simulink model "Control_try"  (R2021b)
settings: Solver=VariableStepAuto  StartTime=0.0  StopTime=inf  RelTol=1e-3
undefined symbols (not defined in the file or in its folder): DiscIntNeverNeededParam
libraries: mobileRoboticsLib x25, simulink_extras x1
(part 1 of 2)
settings Model: Creator=its_ghani  LastModifiedBy=nitis

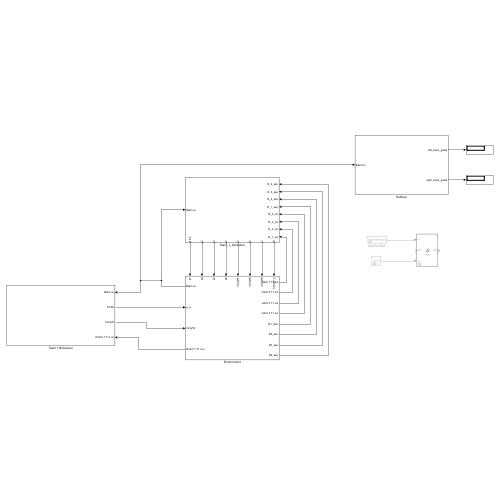
[thumbnail: Simulink's stored preview of the top-level diagram]
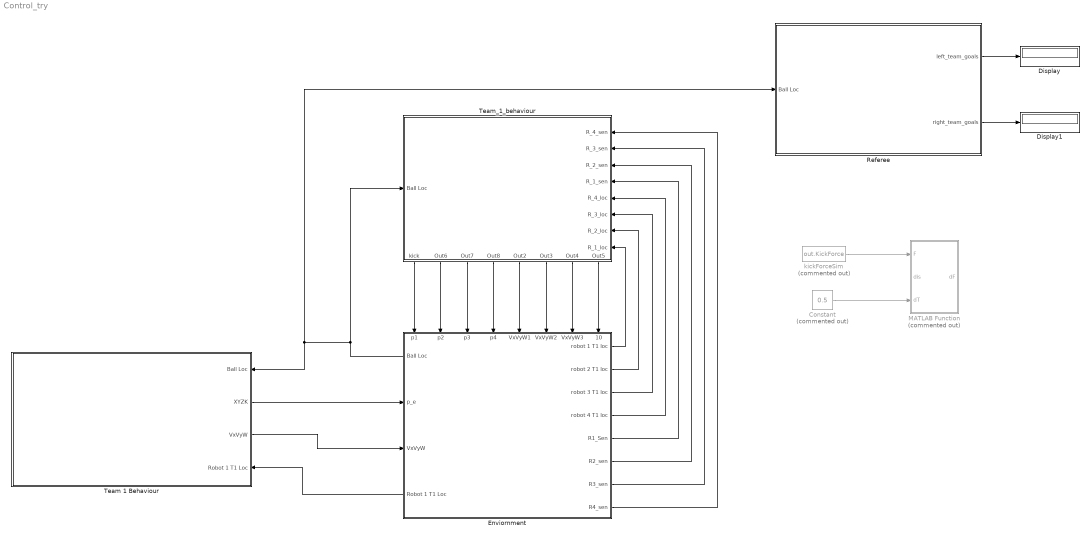
== system Control_try ==
  Constant : Constant  Commented=on  Value=0.5
  Display : Display
  Display1 : Display
  Enviornment : Subsystem
      settings: PortSchema="{\"entries\":[{\"content\":{\"sides\":[{\"content\":{\"connectorIds\":[\"Out9\",\"In1\",\"In2\",\"Out10\"]},\"type\":\"ConnectorPlacement.EquallySpacedRectSide\",\"uuid\":\"bfc4f995-18bb-40a5-813e-439d500b4bf9\"},{\"content\":{\"connectorIds\":[\"Out1\",\"Out2\",\"Out3\",\"Out4\",\"Out5\",\"Out6\",\"Out7\",\"Out8\"],\"side\":\"RIGHT\"},\"type\":\"ConnectorPlacement.EquallySpacedRectSide\",\"uuid\":\"3fb6b8a6-16df-4a59-8ba5-6321e26d1fdd\"},{\"content\":{\"connectorIds\":[\"In3\",\"In4\",\"In5\",\"In6\",\"In7\",\"In8\",\"In9\",\"In10\"],\"side\":\"TOP\"},\"type\":\"ConnectorPlacement.EquallySpacedRectSide\",\"uuid\":\"a9e4cd1b-3afe-4395-99fa-15aef12a4070\"}]},\"type\":\"ConnectorPlacement.EquallySpacedConnector\",\"uuid\":\"a6ca697e-fe67-43ac-b669-91f3e6c836c9\"}],\"packageUris\":[\"http://schema.mathworks.com/mf0/Connector/R2020b\"],\"version\":\"1.0\"}"
  MATLAB Function : MATLAB Function  Commented=on  TreatAsAtomicUnit=on
  Referee : Subsystem
  Team 1 Behaviour : Subsystem
      settings: PortSchema="{\"entries\":[{\"content\":{\"sides\":[{\"content\":{\"connectorIds\":[]},\"type\":\"ConnectorPlacement.EquallySpacedRectSide\",\"uuid\":\"be901545-21b9-45e5-bac5-a8cb9027aef5\"},{\"content\":{\"connectorIds\":[\"In1\",\"Out1\",\"Out2\",\"In2\"],\"side\":\"RIGHT\"},\"type\":\"ConnectorPlacement.EquallySpacedRectSide\",\"uuid\":\"b7c1eb84-2f14-4c7f-a74c-d56efbe0743e\"},{\"content\":{\"connectorIds\":[],\"side\":\"TOP\"},\"type\":\"ConnectorPlacement.EquallySpacedRectSide\",\"uuid\":\"aca41723-ed3f-4bd2-8fc1-457d075e3460\"}]},\"type\":\"ConnectorPlacement.EquallySpacedConnector\",\"uuid\":\"e10e22f1-c8f0-4dfc-85d2-4ba01528372d\"}],\"packageUris\":[\"http://schema.mathworks.com/mf0/Connector/R2020b\"],\"version\":\"1.0\"}"
  Team_1_behaviour : Subsystem
      settings: PortSchema="{\"entries\":[{\"content\":{\"sides\":[{\"content\":{\"connectorIds\":[\"In1\"]},\"type\":\"ConnectorPlacement.EquallySpacedRectSide\",\"uuid\":\"3d238569-03e8-47ba-93af-d09e13fdb2d4\"},{\"content\":{\"connectorIds\":[\"In2\",\"In3\",\"In4\",\"In5\",\"In6\",\"In7\",\"In8\",\"In9\"],\"side\":\"RIGHT\"},\"type\":\"ConnectorPlacement.EquallySpacedRectSide\",\"uuid\":\"12d8afb4-4727-4f82-8566-507ab080c6de\"},{\"content\":{\"connectorIds\":[],\"side\":\"TOP\"},\"type\":\"ConnectorPlacement.EquallySpacedRectSide\",\"uuid\":\"c52fa7ec-51b7-43be-84ca-6ce417c012c7\"},{\"content\":{\"connectorIds\":[\"Out1\",\"Out2\",\"Out3\",\"Out4\",\"Out5\",\"Out6\",\"Out7\",\"Out8\"],\"side\":\"BOTTOM\"},\"type\":\"ConnectorPlacement.EquallySpacedRectSide\",\"uuid\":\"1ba4ac49-8e90-4b3f-8374-c14756940453\"}]},\"type\":\"ConnectorPlacement.EquallySpacedConnector\",\"uuid\":\"883bb5df-d6b2-498f-94a4-3b94e28c6a8f\"}],\"packageUris\":[\"http://schema.mathworks.com/mf0/Connector/R2020b\"],\"version\":\"1.0\"}"
  kickForceSim : FromWorkspace  Commented=on  VariableName=out.KickForce
  wires:
  Enviornment/9(Ball Loc) -> Team_1_behaviour/1(Ball Loc), Referee/1(Ball Loc), Team 1 Behaviour/1(Ball Loc)
  Team 1 Behaviour/1(XYZK) -> Enviornment/1(p_e)
  Referee/2(right_team_goals) -> Display1/1
  Referee/1(left_team_goals) -> Display/1
  Team 1 Behaviour/2(VxVyW) -> Enviornment/2(VxVyW)
  Enviornment/10(Robot 1 T1 Loc) -> Team 1 Behaviour/2(Robot 1 T1 Loc)
  Team_1_behaviour/5(Out2) -> Enviornment/7(VxVyW1)
  Team_1_behaviour/6(Out3) -> Enviornment/8(VxVyW2)
  Team_1_behaviour/7(Out4) -> Enviornment/9(VxVyW3)
  Team_1_behaviour/8(Out5) -> Enviornment/10(VxVyW_4)
  Enviornment/1(robot 1 T1 loc) -> Team_1_behaviour/9(R_1_loc)
  Enviornment/2(robot 2 T1 loc) -> Team_1_behaviour/8(R_2_loc)
  Enviornment/3(robot 3 T1 loc) -> Team_1_behaviour/7(R_3_loc)
  Enviornment/4(robot 4 T1 loc) -> Team_1_behaviour/6(R_4_loc)
  Enviornment/5(R1_Sen) -> Team_1_behaviour/5(R_1_sen)
  Enviornment/6(R2_sen) -> Team_1_behaviour/4(R_2_sen)
  Enviornment/7(R3_sen) -> Team_1_behaviour/3(R_3_sen)
  Enviornment/8(R4_sen) -> Team_1_behaviour/2(R_4_sen)
  Team_1_behaviour/1(kick) -> Enviornment/3(p1)
  Team_1_behaviour/2(Out6) -> Enviornment/4(p2)
  Team_1_behaviour/3(Out7) -> Enviornment/5(p3)
  Team_1_behaviour/4(Out8) -> Enviornment/6(p4)
  kickForceSim/1 -> MATLAB Function/1(F)
  Constant/1 -> MATLAB Function/3(dT)

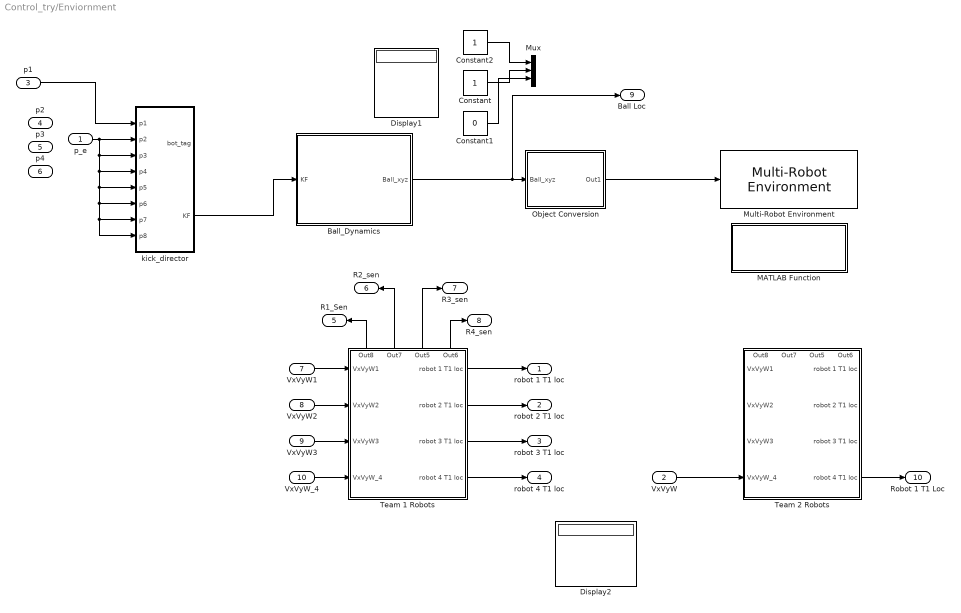
== system Control_try/Enviornment ==
  p_e : Inport
  VxVyW : Inport  Port=2
  p1 : Inport  Port=3
  p2 : Inport  Port=4
  p3 : Inport  Port=5
  p4 : Inport  Port=6
  VxVyW1 : Inport  Port=7
  VxVyW2 : Inport  Port=8
  VxVyW3 : Inport  Port=9
  VxVyW_4 : Inport  Port=10
  "\tTeam 1 Robots" : Subsystem
      settings: PortSchema="{\"entries\":[{\"content\":{\"sides\":[{\"content\":{\"connectorIds\":[\"In1\",\"In2\",\"In3\",\"In4\"]},\"type\":\"ConnectorPlacement.EquallySpacedRectSide\",\"uuid\":\"e759642f-fbca-4f1e-b212-daca2c4962f8\"},{\"content\":{\"connectorIds\":[\"Out1\",\"Out2\",\"Out3\",\"Out4\"],\"side\":\"RIGHT\"},\"type\":\"ConnectorPlacement.EquallySpacedRectSide\",\"uuid\":\"6e1699fa-b246-4758-836f-1d4c98857b70\"},{\"content\":{\"connectorIds\":[\"Out5\",\"Out6\",\"Out7\",\"Out8\"],\"side\":\"TOP\"},\"type\":\"ConnectorPlacement.EquallySpacedRectSide\",\"uuid\":\"c1cf0a96-808a-4241-9d01-181cc4ce2a4d\"},{\"content\":{\"connectorIds\":[],\"side\":\"BOTTOM\"},\"type\":\"ConnectorPlacement.EquallySpacedRectSide\",\"uuid\":\"1a7f648f-16d5-4a09-b479-d6590fa53252\"}]},\"type\":\"ConnectorPlacement.EquallySpacedConnector\",\"uuid\":\"5972ed04-ecdd-4117-bf5d-456318b5c4b8\"}],\"packageUris\":[\"http://schema.mathworks.com/mf0/Connector/R2020b\"],\"version\":\"1.0\"}"
  "\tTeam 2 Robots" : Subsystem
      settings: PortSchema="{\"entries\":[{\"content\":{\"sides\":[{\"content\":{\"connectorIds\":[\"In1\",\"In2\",\"In3\",\"In4\"]},\"type\":\"ConnectorPlacement.EquallySpacedRectSide\",\"uuid\":\"e759642f-fbca-4f1e-b212-daca2c4962f8\"},{\"content\":{\"connectorIds\":[\"Out1\",\"Out2\",\"Out3\",\"Out4\"],\"side\":\"RIGHT\"},\"type\":\"ConnectorPlacement.EquallySpacedRectSide\",\"uuid\":\"6e1699fa-b246-4758-836f-1d4c98857b70\"},{\"content\":{\"connectorIds\":[\"Out5\",\"Out6\",\"Out7\",\"Out8\"],\"side\":\"TOP\"},\"type\":\"ConnectorPlacement.EquallySpacedRectSide\",\"uuid\":\"c1cf0a96-808a-4241-9d01-181cc4ce2a4d\"},{\"content\":{\"connectorIds\":[],\"side\":\"BOTTOM\"},\"type\":\"ConnectorPlacement.EquallySpacedRectSide\",\"uuid\":\"1a7f648f-16d5-4a09-b479-d6590fa53252\"}]},\"type\":\"ConnectorPlacement.EquallySpacedConnector\",\"uuid\":\"5972ed04-ecdd-4117-bf5d-456318b5c4b8\"}],\"packageUris\":[\"http://schema.mathworks.com/mf0/Connector/R2020b\"],\"version\":\"1.0\"}"
  Ball_Dynamics : Subsystem
  Constant : Constant
  Constant1 : Constant  Value=0
  Constant2 : Constant
  Display1 : Display
  Display2 : Display
  MATLAB Function : MATLAB Function  TreatAsAtomicUnit=on
  Multi-Robot Environment : mobileRoboticsLib/Environments/Multi-Robot Environment  numRobots=8  showWaypoints=off  showObjects=on  objectColors=[1 0 0;0 1 0;0 0 1]  objectMarkers='c'  showRobotIds=on  plotSensorLines=on
      settings: SourceProductName=Mobile Robotics Simulation Toolbox
  Mux : Mux  Inputs=3
  Object Conversion : Subsystem
  kick_director : Subsystem
  robot 1 T1 loc : Outport
  robot 2 T1 loc : Outport  Port=2
  robot 3 T1 loc : Outport  Port=3
  robot 4 T1 loc : Outport  Port=4
  R1_Sen : Outport  Port=5
  R2_sen : Outport  Port=6
  R3_sen : Outport  Port=7
  R4_sen : Outport  Port=8
  Ball Loc : Outport  Port=9
  Robot 1 T1 Loc : Outport  Port=10
  wires:
  "\tTeam 1 Robots"/1(robot 1 T1 loc) -> robot 1 T1 loc/1
  Object Conversion/1(Out1) -> Multi-Robot Environment/1
  "\tTeam 1 Robots"/2(robot 2 T1 loc) -> robot 2 T1 loc/1
  "\tTeam 1 Robots"/3(robot 3 T1 loc) -> robot 3 T1 loc/1
  "\tTeam 1 Robots"/4(robot 4 T1 loc) -> robot 4 T1 loc/1
  VxVyW1/1 -> "\tTeam 1 Robots"/1(VxVyW1)
  VxVyW3/1 -> "\tTeam 1 Robots"/3(VxVyW3)
  VxVyW_4/1 -> "\tTeam 1 Robots"/4(VxVyW_4)
  "\tTeam 1 Robots"/5(Out8) -> R1_Sen/1
  "\tTeam 1 Robots"/6(Out7) -> R2_sen/1
  "\tTeam 1 Robots"/7(Out5) -> R3_sen/1
  "\tTeam 1 Robots"/8(Out6) -> R4_sen/1
  p_e/1 -> kick_director/4(p4), kick_director/5(p5), kick_director/6(p6), kick_director/7(p7), kick_director/8(p8), kick_director/3(p3), kick_director/2(p2)
  p1/1 -> kick_director/1(p1)
  VxVyW2/1 -> "\tTeam 1 Robots"/2(VxVyW2)
  "\tTeam 2 Robots"/4(robot 4 T1 loc) -> Robot 1 T1 Loc/1
  VxVyW/1 -> "\tTeam 2 Robots"/4(VxVyW_4)
  kick_director/2(KF) -> Ball_Dynamics/1(KF)
  Constant2/1 -> Mux/1
  Constant/1 -> Mux/2
  Constant1/1 -> Mux/3
  Ball_Dynamics/1(Ball_xyz) -> Ball Loc/1, Object Conversion/1(Ball_xyz)

== system Control_try/Referee ==
  Ball Loc : Inport
  Corner : Stateflow chart  TreatAsAtomicUnit=on
  Demux : Demux  Outputs=3
  Display2 : Display
  GOAL : Stateflow chart  TreatAsAtomicUnit=on
  Penelty : Stateflow chart  TreatAsAtomicUnit=on
  Throwin : Stateflow chart  TreatAsAtomicUnit=on
  left_team_goals : Outport
  right_team_goals : Outport  Port=2
  wires:
  Ball Loc/1 -> Display2/1, Demux/1
  Demux/1 -> Throwin/1(X), GOAL/1(X)
  Demux/2 -> Throwin/2(Y), GOAL/2(Y)
  Demux/3 -> GOAL/3(Z)
  GOAL/1(left_team_goal) -> left_team_goals/1
  GOAL/2(right_team_goal) -> right_team_goals/1

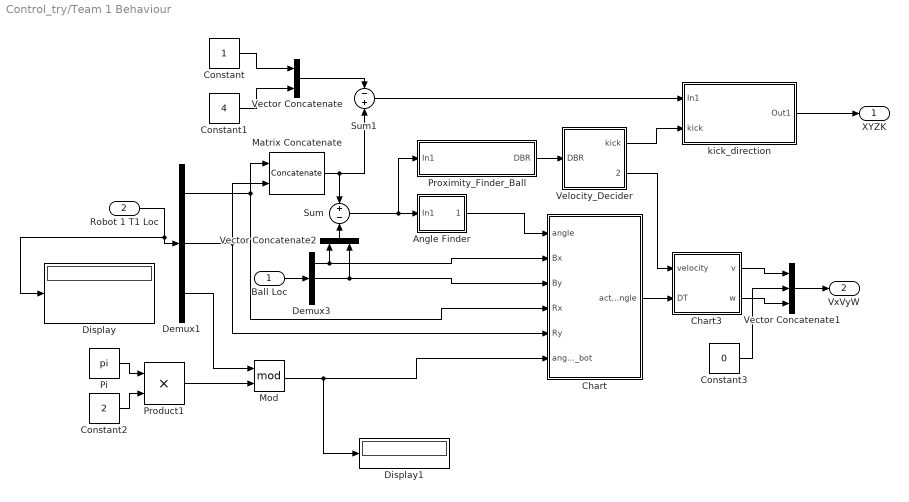
== system Control_try/Team 1 Behaviour ==
  Ball Loc : Inport
  Robot 1 T1 Loc : Inport  Port=2
  Angle Finder : Subsystem
  Chart : Stateflow chart  TreatAsAtomicUnit=on
      settings: PortSchema="{\"entries\":[{\"content\":{\"sides\":[{\"content\":{\"connectorIds\":[\"In5\",\"In1\",\"In2\",\"In3\",\"In4\",\"In6\"]},\"type\":\"ConnectorPlacement.EquallySpacedRectSide\",\"uuid\":\"cd25ea97-6441-4246-83f2-eec847899c89\"},{\"content\":{\"connectorIds\":[\"Out1\"],\"side\":\"RIGHT\"},\"type\":\"ConnectorPlacement.EquallySpacedRectSide\",\"uuid\":\"ef7d77a7-1549-4474-8b84-35bb8af5d0e7\"},{\"content\":{\"connectorIds\":[],\"side\":\"TOP\"},\"type\":\"ConnectorPlacement.EquallySpacedRectSide\",\"uuid\":\"0f0ce596-3061-42ac-890a-62bc4f21ac3e\"},{\"content\":{\"connectorIds\":[],\"side\":\"BOTTOM\"},\"type\":\"ConnectorPlacement.EquallySpacedRectSide\",\"uuid\":\"682b3de5-e999-4954-b7ff-f16ecbf9ea8f\"}]},\"type\":\"ConnectorPlacement.EquallySpacedConnector\",\"uuid\":\"15dca8e2-6a60-4a0d-80a5-3c295a61c828\"}],\"packageUris\":[\"http://schema.mathworks.com/mf0/Connector/R2020b\"],\"version\":\"1.0\"}"
  Chart3 : Stateflow chart  TreatAsAtomicUnit=on
  Constant : Constant
  Constant1 : Constant  Value=4
  Constant2 : Constant  Value=2
  Constant3 : Constant  Value=0
  Demux1 : Demux  Outputs=3
  Demux3 : Demux  Outputs=3
  Display : Display
  Display1 : Display
  Matrix Concatenate : Concatenate  Mode=Multidimensional array  ConcatenateDimension=2
  Mod : Math  Operator=mod  SaturateOnIntegerOverflow=on
  Pi : Constant  Value=pi  OutDataTypeStr=Inherit: Inherit via back propagation
  Product1 : Product
  Proximity_Finder_Ball : Subsystem
  Sum : Sum  Inputs=+-
  Sum1 : Sum  Inputs=-+
  Vector Concatenate : Concatenate
  Vector Concatenate1 : Concatenate  NumInputs=3
  Vector Concatenate2 : Concatenate
  Velocity_Decider : Stateflow chart  TreatAsAtomicUnit=on
  kick_direction : Subsystem
  XYZK : Outport
  VxVyW : Outport  Port=2
  wires:
  Ball Loc/1 -> Demux3/1
  Sum/1 -> Proximity_Finder_Ball/1(In1), Angle Finder/1(In1)
  Robot 1 T1 Loc/1 -> Display/1, Demux1/1
  Demux1/1 -> Matrix Concatenate/1, Chart/3(Rx)
  Demux1/2 -> Matrix Concatenate/2, Chart/4(Ry)
  Matrix Concatenate/1 -> Sum1/2, Sum/1
  Demux3/2 -> Vector Concatenate2/2, Chart/2(By)
  Demux3/1 -> Vector Concatenate2/1, Chart/1(Bx)
  Demux1/3 -> Mod/1
  Pi/1 -> Product1/1
  Constant2/1 -> Product1/2
  Product1/1 -> Mod/2
  Chart/1(actual_angle) -> Chart3/2(DT)
  Mod/1 -> Display1/1, Chart/6(angle_bot)
  Angle Finder/1(angle) -> Chart/5(angle)
  Proximity_Finder_Ball/1(DBR) -> Velocity_Decider/1(DBR)
  Velocity_Decider/2(velocity) -> Chart3/1(velocity)
  Constant/1 -> Vector Concatenate/1
  Constant1/1 -> Vector Concatenate/2
  Vector Concatenate/1 -> Sum1/1
  Sum1/1 -> kick_direction/1(In1)
  Velocity_Decider/1(kick) -> kick_direction/2(kick)
  kick_direction/1(Out1) -> XYZK/1
  Chart3/1(v) -> Vector Concatenate1/1
  Chart3/2(w) -> Vector Concatenate1/3
  Constant3/1 -> Vector Concatenate1/2
  Vector Concatenate1/1 -> VxVyW/1
  Vector Concatenate2/1 -> Sum/2

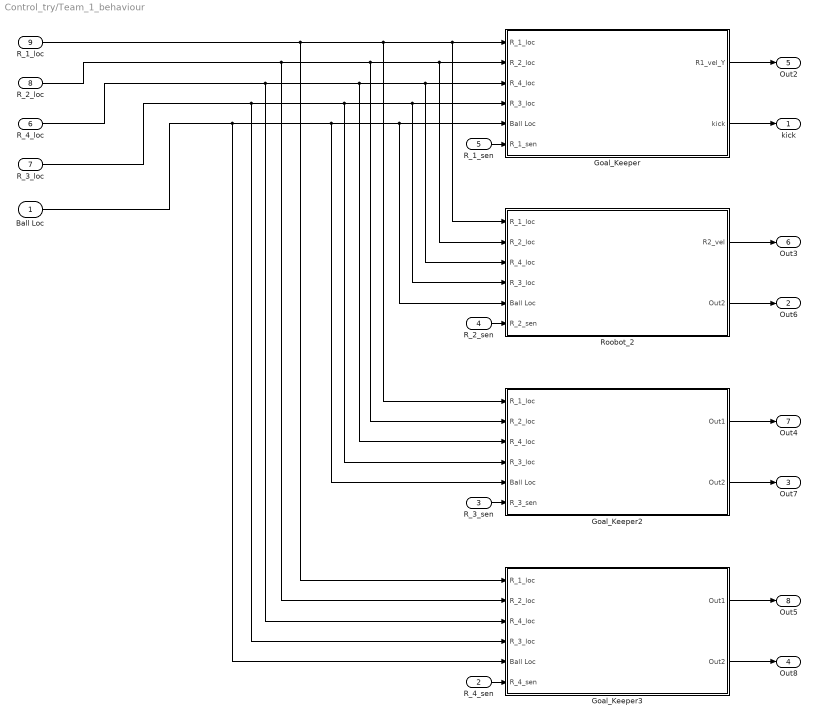
== system Control_try/Team_1_behaviour ==
  Ball Loc : Inport
  R_4_sen : Inport  Port=2
  R_3_sen : Inport  Port=3
  R_2_sen : Inport  Port=4
  R_1_sen : Inport  Port=5
  R_4_loc : Inport  Port=6
  R_3_loc : Inport  Port=7
  R_2_loc : Inport  Port=8
  R_1_loc : Inport  Port=9
  Goal_Keeper : Subsystem
  Goal_Keeper2 : Subsystem
  Goal_Keeper3 : Subsystem
  Roobot_2 : Subsystem
  kick : Outport
  Out6 : Outport  Port=2
  Out7 : Outport  Port=3
  Out8 : Outport  Port=4
  Out2 : Outport  Port=5
  Out3 : Outport  Port=6
  Out4 : Outport  Port=7
  Out5 : Outport  Port=8
  wires:
  Goal_Keeper/1(R1_vel_Y) -> Out2/1
  R_1_sen/1 -> Goal_Keeper/6(R_1_sen)
  R_1_loc/1 -> Goal_Keeper3/1(R_1_loc), Goal_Keeper2/1(R_1_loc), Roobot_2/1(R_1_loc), Goal_Keeper/1(R_1_loc)
  R_2_loc/1 -> Goal_Keeper3/2(R_2_loc), Goal_Keeper2/2(R_2_loc), Roobot_2/2(R_2_loc), Goal_Keeper/2(R_2_loc)
  R_4_loc/1 -> Goal_Keeper3/3(R_4_loc), Goal_Keeper2/3(R_4_loc), Roobot_2/3(R_4_loc), Goal_Keeper/3(R_4_loc)
  R_3_loc/1 -> Goal_Keeper3/4(R_3_loc), Goal_Keeper2/4(R_3_loc), Roobot_2/4(R_3_loc), Goal_Keeper/4(R_3_loc)
  Ball Loc/1 -> Goal_Keeper3/5(Ball Loc), Goal_Keeper2/5(Ball Loc), Roobot_2/5(Ball Loc), Goal_Keeper/5(Ball Loc)
  R_2_sen/1 -> Roobot_2/6(R_2_sen)
  R_3_sen/1 -> Goal_Keeper2/6(R_3_sen)
  R_4_sen/1 -> Goal_Keeper3/6(R_4_sen)
  Roobot_2/1(R2_vel) -> Out3/1
  Goal_Keeper2/1(Out1) -> Out4/1
  Goal_Keeper3/1(Out1) -> Out5/1
  Goal_Keeper/2(kick) -> kick/1
  Roobot_2/2(Out2) -> Out6/1
  Goal_Keeper2/2(Out2) -> Out7/1
  Goal_Keeper3/2(Out2) -> Out8/1

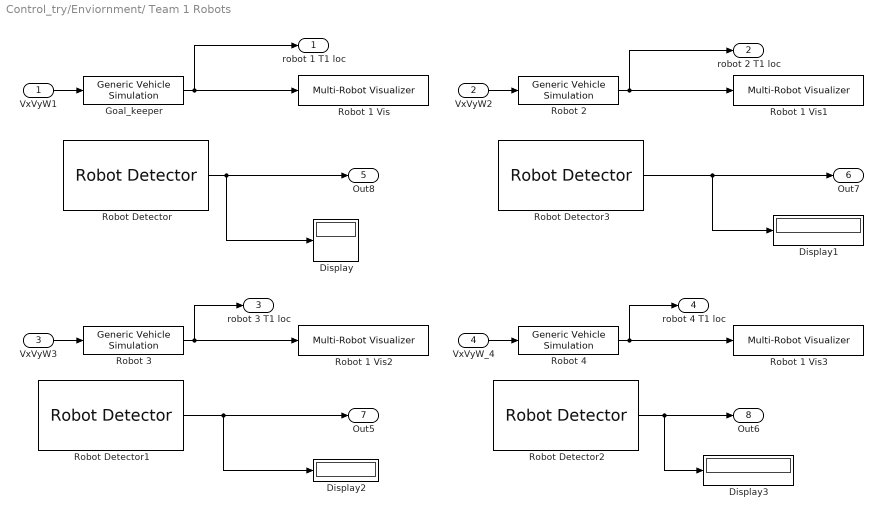
== system Control_try/Enviornment/	Team 1 Robots ==
  VxVyW1 : Inport
  VxVyW2 : Inport  Port=2
  VxVyW3 : Inport  Port=3
  VxVyW_4 : Inport  Port=4
  Display{,1..3} (4 alike) : Display
  Goal_keeper : mobileRoboticsLib/Utilities/Generic Vehicle Simulation  initX=1.5  initY=4  initAngle=0  Ts=0.05
      settings: SourceProductName=Mobile Robotics Simulation Toolbox
  Robot 1 Vis : mobileRoboticsLib/Environments/Multi-Robot Visualizer  idx=1  radius=0.5  robotColor=[0 0 1]  showTraj=on  hasLidar=off  sensorOffset=[0,0]  scanAngles=[-pi/4, 0, pi/4]  hasObjDetector=off  objDetectorOffset=[0,0]  objDetectorAngle=0  objDetectorFOV=pi/3  objDetectorMaxRange=5
      settings: SourceProductName=Mobile Robotics Simulation Toolbox
  Robot 1 Vis1 : mobileRoboticsLib/Environments/Multi-Robot Visualizer  idx=2  radius=0.5  robotColor=[0 0 1]  showTraj=on  hasLidar=off  sensorOffset=[0,0]  scanAngles=[-pi/4, 0, pi/4]  hasObjDetector=off  objDetectorOffset=[0,0]  objDetectorAngle=0  objDetectorFOV=pi/3  objDetectorMaxRange=5
      settings: SourceProductName=Mobile Robotics Simulation Toolbox
  Robot 1 Vis2 : mobileRoboticsLib/Environments/Multi-Robot Visualizer  idx=3  radius=0.5  robotColor=[0 0 1]  showTraj=on  hasLidar=off  sensorOffset=[0,0]  scanAngles=[-pi/4, 0, pi/4]  hasObjDetector=off  objDetectorOffset=[0,0]  objDetectorAngle=0  objDetectorFOV=pi/3  objDetectorMaxRange=5
      settings: SourceProductName=Mobile Robotics Simulation Toolbox
  Robot 1 Vis3 : mobileRoboticsLib/Environments/Multi-Robot Visualizer  idx=4  radius=0.5  robotColor=[0 0 1]  showTraj=on  hasLidar=off  sensorOffset=[0,0]  scanAngles=[-pi/4, 0, pi/4]  hasObjDetector=off  objDetectorOffset=[0,0]  objDetectorAngle=0  objDetectorFOV=pi/3  objDetectorMaxRange=5
      settings: SourceProductName=Mobile Robotics Simulation Toolbox
  Robot 2 : mobileRoboticsLib/Utilities/Generic Vehicle Simulation  initX=3.25  initY=2.5  initAngle=0  Ts=0.05
      settings: SourceProductName=Mobile Robotics Simulation Toolbox
  Robot 3 : mobileRoboticsLib/Utilities/Generic Vehicle Simulation  initX=3.25  initY=5.5  initAngle=0  Ts=0.05
      settings: SourceProductName=Mobile Robotics Simulation Toolbox
  Robot 4 : mobileRoboticsLib/Utilities/Generic Vehicle Simulation  initX=5.25  initY=4.25  initAngle=0  Ts=0.05
      settings: SourceProductName=Mobile Robotics Simulation Toolbox
  Robot Detector : mobileRoboticsLib/Environments/Robot Detector  robotIdx=1  sensorOffset=[ 0, 0 ]  sensorAngle=0  fieldOfView=pi/3  maxRange=3  maxDetections=7  sampleTime=0.1
      settings: SourceProductName=Mobile Robotics Simulation Toolbox
  Robot Detector1 : mobileRoboticsLib/Environments/Robot Detector  robotIdx=3  sensorOffset=[ 0, 0 ]  sensorAngle=0  fieldOfView=pi/3  maxRange=1.5  maxDetections=7  sampleTime=0.1
      settings: SourceProductName=Mobile Robotics Simulation Toolbox
  Robot Detector2 : mobileRoboticsLib/Environments/Robot Detector  robotIdx=4  sensorOffset=[ 0, 0 ]  sensorAngle=0  fieldOfView=pi/3  maxRange=1.5  maxDetections=7  sampleTime=0.1
      settings: SourceProductName=Mobile Robotics Simulation Toolbox
  Robot Detector3 : mobileRoboticsLib/Environments/Robot Detector  robotIdx=2  sensorOffset=[ 0, 0 ]  sensorAngle=0  fieldOfView=pi/3  maxRange=1.5  maxDetections=7  sampleTime=0.1
      settings: SourceProductName=Mobile Robotics Simulation Toolbox
  robot 1 T1 loc : Outport
  robot 2 T1 loc : Outport  Port=2
  robot 3 T1 loc : Outport  Port=3
  robot 4 T1 loc : Outport  Port=4
  Out8 : Outport  Port=5
  Out7 : Outport  Port=6
  Out5 : Outport  Port=7
  Out6 : Outport  Port=8
  wires:
  Goal_keeper/1 -> robot 1 T1 loc/1, Robot 1 Vis/1
  VxVyW1/1 -> Goal_keeper/1
  VxVyW2/1 -> Robot 2/1
  Robot 2/1 -> robot 2 T1 loc/1, Robot 1 Vis1/1
  Robot 3/1 -> Robot 1 Vis2/1, robot 3 T1 loc/1
  VxVyW3/1 -> Robot 3/1
  VxVyW_4/1 -> Robot 4/1
  Robot 4/1 -> robot 4 T1 loc/1, Robot 1 Vis3/1
  Robot Detector3/1 -> Out7/1, Display1/1
  Robot Detector1/1 -> Out5/1, Display2/1
  Robot Detector2/1 -> Out6/1, Display3/1
  Robot Detector/1 -> Display/1, Out8/1

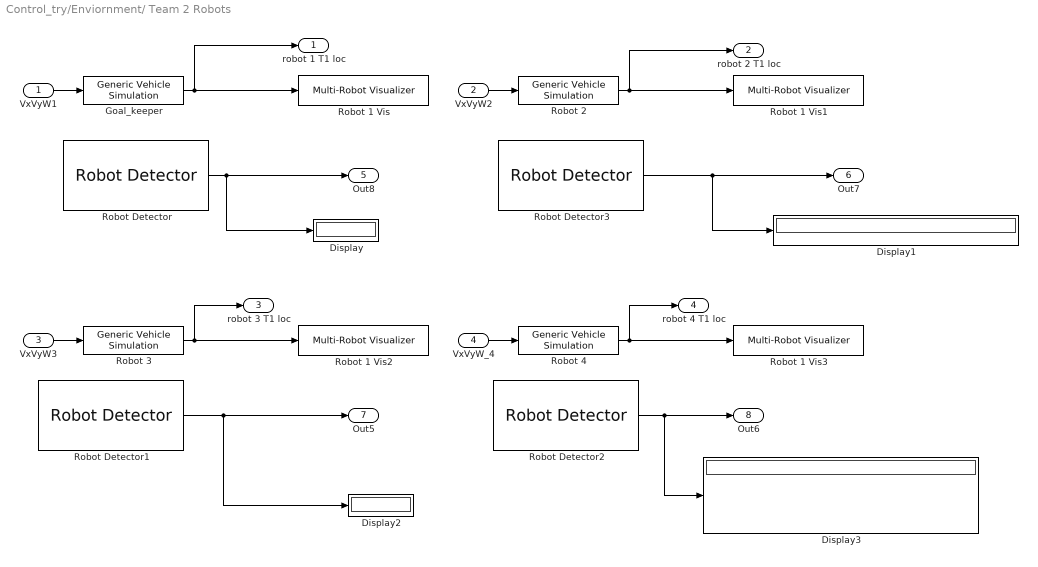
== system Control_try/Enviornment/	Team 2 Robots ==
  VxVyW1 : Inport
  VxVyW2 : Inport  Port=2
  VxVyW3 : Inport  Port=3
  VxVyW_4 : Inport  Port=4
  Display{,1..3} (4 alike) : Display
  Goal_keeper : mobileRoboticsLib/Utilities/Generic Vehicle Simulation  initX=9.5  initY=4  initAngle=pi  Ts=0.05
      settings: SourceProductName=Mobile Robotics Simulation Toolbox
  Robot 1 Vis : mobileRoboticsLib/Environments/Multi-Robot Visualizer  idx=5  radius=0.5  robotColor=[1 0 0]  showTraj=on  hasLidar=off  sensorOffset=[0,0]  scanAngles=[-pi/4, 0, pi/4]  hasObjDetector=off  objDetectorOffset=[0,0]  objDetectorAngle=0  objDetectorFOV=pi/3  objDetectorMaxRange=5
      settings: SourceProductName=Mobile Robotics Simulation Toolbox
  Robot 1 Vis1 : mobileRoboticsLib/Environments/Multi-Robot Visualizer  idx=6  radius=0.5  robotColor=[0.1 1 1]  showTraj=on  hasLidar=off  sensorOffset=[0,0]  scanAngles=[-pi/4, 0, pi/4]  hasObjDetector=off  objDetectorOffset=[0,0]  objDetectorAngle=0  objDetectorFOV=pi/3  objDetectorMaxRange=5
      settings: SourceProductName=Mobile Robotics Simulation Toolbox
  Robot 1 Vis2 : mobileRoboticsLib/Environments/Multi-Robot Visualizer  idx=7  radius=0.5  robotColor=[0 1 1]  showTraj=on  hasLidar=off  sensorOffset=[0,0]  scanAngles=[-pi/4, 0, pi/4]  hasObjDetector=off  objDetectorOffset=[0,0]  objDetectorAngle=0  objDetectorFOV=pi/3  objDetectorMaxRange=5
      settings: SourceProductName=Mobile Robotics Simulation Toolbox
  Robot 1 Vis3 : mobileRoboticsLib/Environments/Multi-Robot Visualizer  idx=8  radius=0.5  robotColor=[0 1 1]  showTraj=on  hasLidar=off  sensorOffset=[0,0]  scanAngles=[-pi/4, 0, pi/4]  hasObjDetector=off  objDetectorOffset=[0,0]  objDetectorAngle=0  objDetectorFOV=pi/3  objDetectorMaxRange=5
      settings: SourceProductName=Mobile Robotics Simulation Toolbox
  Robot 2 : mobileRoboticsLib/Utilities/Generic Vehicle Simulation  initX=3.5  initY=4  initAngle=pi  Ts=0.05
      settings: SourceProductName=Mobile Robotics Simulation Toolbox
  Robot 3 : mobileRoboticsLib/Utilities/Generic Vehicle Simulation  initX=3.5  initY=3.5  initAngle=pi  Ts=0.05
      settings: SourceProductName=Mobile Robotics Simulation Toolbox
  Robot 4 : mobileRoboticsLib/Utilities/Generic Vehicle Simulation  initX=7.75  initY=2.5  initAngle=pi  Ts=0.05
      settings: SourceProductName=Mobile Robotics Simulation Toolbox
  Robot Detector : mobileRoboticsLib/Environments/Robot Detector  robotIdx=5  sensorOffset=[ 0, 0 ]  sensorAngle=0  fieldOfView=pi/3  maxRange=1.5  maxDetections=7  sampleTime=0.1
      settings: SourceProductName=Mobile Robotics Simulation Toolbox
  Robot Detector1 : mobileRoboticsLib/Environments/Robot Detector  robotIdx=7  sensorOffset=[ 0, 0 ]  sensorAngle=0  fieldOfView=pi/3  maxRange=1.5  maxDetections=7  sampleTime=0.1
      settings: SourceProductName=Mobile Robotics Simulation Toolbox
  Robot Detector2 : mobileRoboticsLib/Environments/Robot Detector  robotIdx=8  sensorOffset=[ 0, 0 ]  sensorAngle=0  fieldOfView=pi/3  maxRange=1.5  maxDetections=7  sampleTime=0.1
      settings: SourceProductName=Mobile Robotics Simulation Toolbox
  Robot Detector3 : mobileRoboticsLib/Environments/Robot Detector  robotIdx=6  sensorOffset=[ 0, 0 ]  sensorAngle=0  fieldOfView=pi/3  maxRange=1.5  maxDetections=7  sampleTime=0.1
      settings: SourceProductName=Mobile Robotics Simulation Toolbox
  robot 1 T1 loc : Outport
  robot 2 T1 loc : Outport  Port=2
  robot 3 T1 loc : Outport  Port=3
  robot 4 T1 loc : Outport  Port=4
  Out8 : Outport  Port=5
  Out7 : Outport  Port=6
  Out5 : Outport  Port=7
  Out6 : Outport  Port=8
  wires:
  Goal_keeper/1 -> robot 1 T1 loc/1, Robot 1 Vis/1
  VxVyW1/1 -> Goal_keeper/1
  VxVyW2/1 -> Robot 2/1
  Robot 2/1 -> robot 2 T1 loc/1, Robot 1 Vis1/1
  Robot 3/1 -> Robot 1 Vis2/1, robot 3 T1 loc/1
  VxVyW3/1 -> Robot 3/1
  VxVyW_4/1 -> Robot 4/1
  Robot 4/1 -> robot 4 T1 loc/1, Robot 1 Vis3/1
  Robot Detector3/1 -> Out7/1, Display1/1
  Robot Detector1/1 -> Out5/1, Display2/1
  Robot Detector2/1 -> Out6/1, Display3/1
  Robot Detector/1 -> Display/1, Out8/1

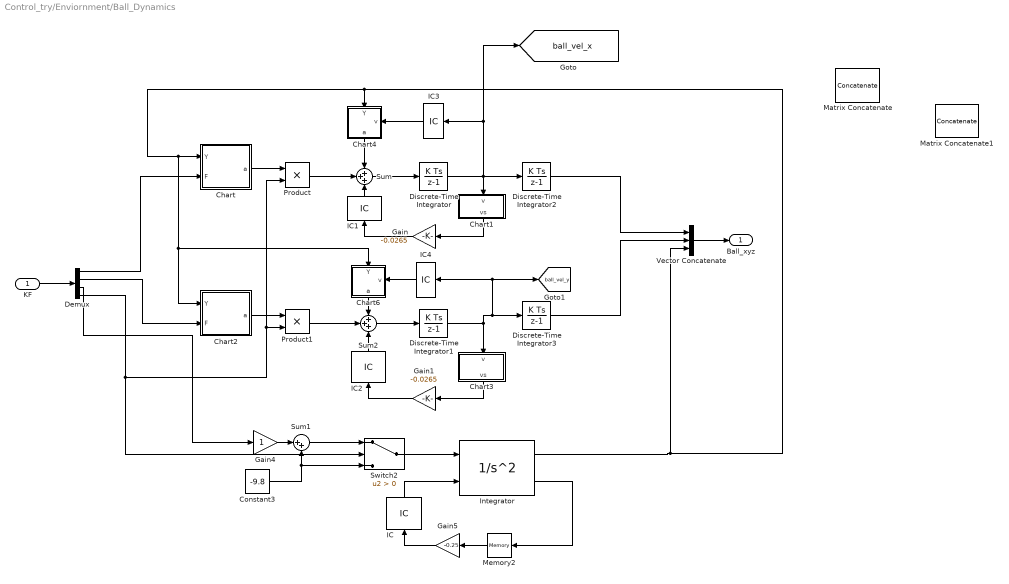
== system Control_try/Enviornment/Ball_Dynamics ==
  KF : Inport
  Chart : Stateflow chart  TreatAsAtomicUnit=on
  Chart1 : Stateflow chart  TreatAsAtomicUnit=on
      settings: PortSchema="{\"entries\":[{\"content\":{\"sides\":[{\"content\":{\"connectorIds\":[]},\"type\":\"ConnectorPlacement.EquallySpacedRectSide\",\"uuid\":\"edcb69b6-c92b-474e-86d7-1e52c2e82b28\"},{\"content\":{\"connectorIds\":[],\"side\":\"RIGHT\"},\"type\":\"ConnectorPlacement.EquallySpacedRectSide\",\"uuid\":\"df9771e4-6870-4305-9c84-3f71fcb76e6b\"},{\"content\":{\"connectorIds\":[\"In1\"],\"side\":\"TOP\"},\"type\":\"ConnectorPlacement.EquallySpacedRectSide\",\"uuid\":\"56b80241-156d-4669-9174-884a577f2013\"},{\"content\":{\"connectorIds\":[\"Out1\"],\"side\":\"BOTTOM\"},\"type\":\"ConnectorPlacement.EquallySpacedRectSide\",\"uuid\":\"179af6a7-cab5-4faa-a562-268e2d2e4d3e\"}]},\"type\":\"ConnectorPlacement.EquallySpacedConnector\",\"uuid\":\"707001f1-02b8-4f5e-ba3f-f155c99072e5\"}],\"packageUris\":[\"http://schema.mathworks.com/mf0/Connector/R2020b\"],\"version\":\"1.0\"}"
  Chart2 : Stateflow chart  TreatAsAtomicUnit=on
  Chart3 : Stateflow chart  TreatAsAtomicUnit=on
      settings: PortSchema="{\"entries\":[{\"content\":{\"sides\":[{\"content\":{\"connectorIds\":[]},\"type\":\"ConnectorPlacement.EquallySpacedRectSide\",\"uuid\":\"edcb69b6-c92b-474e-86d7-1e52c2e82b28\"},{\"content\":{\"connectorIds\":[],\"side\":\"RIGHT\"},\"type\":\"ConnectorPlacement.EquallySpacedRectSide\",\"uuid\":\"df9771e4-6870-4305-9c84-3f71fcb76e6b\"},{\"content\":{\"connectorIds\":[\"In1\"],\"side\":\"TOP\"},\"type\":\"ConnectorPlacement.EquallySpacedRectSide\",\"uuid\":\"56b80241-156d-4669-9174-884a577f2013\"},{\"content\":{\"connectorIds\":[\"Out1\"],\"side\":\"BOTTOM\"},\"type\":\"ConnectorPlacement.EquallySpacedRectSide\",\"uuid\":\"179af6a7-cab5-4faa-a562-268e2d2e4d3e\"}]},\"type\":\"ConnectorPlacement.EquallySpacedConnector\",\"uuid\":\"707001f1-02b8-4f5e-ba3f-f155c99072e5\"}],\"packageUris\":[\"http://schema.mathworks.com/mf0/Connector/R2020b\"],\"version\":\"1.0\"}"
  Chart4 : Stateflow chart  TreatAsAtomicUnit=on
      settings: PortSchema="{\"entries\":[{\"content\":{\"sides\":[{\"content\":{\"connectorIds\":[]},\"type\":\"ConnectorPlacement.EquallySpacedRectSide\",\"uuid\":\"edcb69b6-c92b-474e-86d7-1e52c2e82b28\"},{\"content\":{\"connectorIds\":[\"In2\"],\"side\":\"RIGHT\"},\"type\":\"ConnectorPlacement.EquallySpacedRectSide\",\"uuid\":\"df9771e4-6870-4305-9c84-3f71fcb76e6b\"},{\"content\":{\"connectorIds\":[\"In1\"],\"side\":\"TOP\"},\"type\":\"ConnectorPlacement.EquallySpacedRectSide\",\"uuid\":\"56b80241-156d-4669-9174-884a577f2013\"},{\"content\":{\"connectorIds\":[\"Out1\"],\"side\":\"BOTTOM\"},\"type\":\"ConnectorPlacement.EquallySpacedRectSide\",\"uuid\":\"6d9abc99-74e1-40c2-a49f-e0d9410a29cc\"}]},\"type\":\"ConnectorPlacement.EquallySpacedConnector\",\"uuid\":\"707001f1-02b8-4f5e-ba3f-f155c99072e5\"}],\"packageUris\":[\"http://schema.mathworks.com/mf0/Connector/R2020b\"],\"version\":\"1.0\"}"
  Chart6 : Stateflow chart  TreatAsAtomicUnit=on
      settings: PortSchema="{\"entries\":[{\"content\":{\"sides\":[{\"content\":{\"connectorIds\":[]},\"type\":\"ConnectorPlacement.EquallySpacedRectSide\",\"uuid\":\"edcb69b6-c92b-474e-86d7-1e52c2e82b28\"},{\"content\":{\"connectorIds\":[\"In2\"],\"side\":\"RIGHT\"},\"type\":\"ConnectorPlacement.EquallySpacedRectSide\",\"uuid\":\"df9771e4-6870-4305-9c84-3f71fcb76e6b\"},{\"content\":{\"connectorIds\":[\"In1\"],\"side\":\"TOP\"},\"type\":\"ConnectorPlacement.EquallySpacedRectSide\",\"uuid\":\"56b80241-156d-4669-9174-884a577f2013\"},{\"content\":{\"connectorIds\":[\"Out1\"],\"side\":\"BOTTOM\"},\"type\":\"ConnectorPlacement.EquallySpacedRectSide\",\"uuid\":\"6d9abc99-74e1-40c2-a49f-e0d9410a29cc\"}]},\"type\":\"ConnectorPlacement.EquallySpacedConnector\",\"uuid\":\"707001f1-02b8-4f5e-ba3f-f155c99072e5\"}],\"packageUris\":[\"http://schema.mathworks.com/mf0/Connector/R2020b\"],\"version\":\"1.0\"}"
  Constant3 : Constant  Value=-9.8
  Demux : Demux
  Discrete-Time Integrator : DiscreteIntegrator  SampleTime=-1  ICPrevOutput=DiscIntNeverNeededParam  ICPrevScaledInput=DiscIntNeverNeededParam
  Discrete-Time Integrator1 : DiscreteIntegrator  SampleTime=-1  ICPrevOutput=DiscIntNeverNeededParam  ICPrevScaledInput=DiscIntNeverNeededParam
  Discrete-Time Integrator2 : DiscreteIntegrator  InitialCondition=5.5  SampleTime=-1  ICPrevOutput=DiscIntNeverNeededParam  ICPrevScaledInput=DiscIntNeverNeededParam
  Discrete-Time Integrator3 : DiscreteIntegrator  InitialCondition=4  SampleTime=-1  ICPrevOutput=DiscIntNeverNeededParam  ICPrevScaledInput=DiscIntNeverNeededParam
  Gain : Gain  Gain=-0.0265
  Gain1 : Gain  Gain=-0.0265
  Gain4 : Gain
  Gain5 : Gain  Gain=-0.25
  IC : InitialCondition
  IC{1..4} (4 alike) : InitialCondition  Value=0
  Integrator : SecondOrderIntegrator  ICX=0  LimitX=on  LowerLimitX=0.0  StateNameX='Position'  ICSourceDXDT=external  StateNameDXDT='Velocity'  ReinitDXDTwhenXreachesSaturation=on
  Matrix Concatenate : Concatenate  Mode=Multidimensional array  ConcatenateDimension=2
  Matrix Concatenate1 : Concatenate  Mode=Multidimensional array  ConcatenateDimension=2
  Memory2 : Memory
  Product : Product
  Product1 : Product
  Sum : Sum  Inputs=+++
  Sum1 : Sum  Inputs=|++
  Sum2 : Sum  Inputs=+++
  Switch2 : Switch  Criteria=u2 > Threshold
  Vector Concatenate : Concatenate  NumInputs=3
  Ball_xyz : Outport
  tag scope: ball_vel_x=global, ball_vel_y=global
  wires:
  Constant3/1 -> Sum1/2, Switch2/3
  Integrator/2 -> Memory2/1
  Memory2/1 -> Gain5/1
  IC/1 -> Integrator/2
  Switch2/1 -> Integrator/1
  Sum1/1 -> Switch2/1
  Gain4/1 -> Sum1/1
  Demux/3 -> Gain4/1
  Demux/4 -> Switch2/2, Product/2, Product1/2
  Gain5/1 -> IC/1
  KF/1 -> Demux/1
  Gain/1 -> IC1/1
  Chart/1(a) -> Product/1
  Sum/1 -> Discrete-Time Integrator/1
  Discrete-Time Integrator1/1 -> [ball_vel_y], IC4/1, Discrete-Time Integrator3/1, Chart3/1(v)
  Chart2/1(a) -> Product1/1
  Gain1/1 -> IC2/1
  Product1/1 -> Sum2/2
  Sum2/1 -> Discrete-Time Integrator1/1
  Demux/1 -> Chart/2(F)
  Demux/2 -> Chart2/2(F)
  Integrator/1 -> Vector Concatenate/3, Chart6/1(Y), Chart2/1(Y), Chart/1(Y), Chart4/1(Y)
  Chart1/1(vs) -> Gain/1
  Chart3/1(vs) -> Gain1/1
  IC3/1 -> Chart4/2(v)
  Discrete-Time Integrator/1 -> [ball_vel_x], IC3/1, Discrete-Time Integrator2/1, Chart1/1(v)
  Product/1 -> Sum/2
  IC2/1 -> Sum2/3
  IC1/1 -> Sum/3
  IC4/1 -> Chart6/2(v)
  Chart4/1(a) -> Sum/1
  Chart6/1(a) -> Sum2/1
  Vector Concatenate/1 -> Ball_xyz/1
  Discrete-Time Integrator2/1 -> Vector Concatenate/1
  Discrete-Time Integrator3/1 -> Vector Concatenate/2

== system Control_try/Enviornment/Object Conversion ==
  Ball_xyz : Inport
  Ball : Constant
  Demux : Demux  Outputs=3
  Matrix Concatenate : Concatenate  NumInputs=3  Mode=Multidimensional array  ConcatenateDimension=2
  Out1 : Outport
  wires:
  Ball/1 -> Matrix Concatenate/3
  Matrix Concatenate/1 -> Out1/1
  Ball_xyz/1 -> Demux/1
  Demux/1 -> Matrix Concatenate/1
  Demux/2 -> Matrix Concatenate/2

== system Control_try/Enviornment/kick_director ==
  p1 : Inport
  p2 : Inport  Port=2
  p3 : Inport  Port=3
  p4 : Inport  Port=4
  p5 : Inport  Port=5
  p6 : Inport  Port=6
  p7 : Inport  Port=7
  p8 : Inport  Port=8
  Chart : Stateflow chart  TreatAsAtomicUnit=on
  To Workspace1 : ToWorkspace  VariableName=simout1  SaveFormat=Timeseries  SampleTime=-1
  bot_tag : Outport
  KF : Outport  Port=2
  wires:
  Chart/2(KF) -> KF/1
  Chart/1(bot_tag) -> bot_tag/1
  p1/1 -> To Workspace1/1, Chart/1(p1)
  p2/1 -> Chart/2(p2)
  p3/1 -> Chart/3(p3)
  p4/1 -> Chart/4(p4)
  p5/1 -> Chart/5(p5)
  p6/1 -> Chart/6(p6)
  p7/1 -> Chart/7(p7)
  p8/1 -> Chart/8(p8)

== system Control_try/Team 1 Behaviour/Angle Finder ==
  In1 : Inport
  Abs : Abs
  Atan : Trigonometry  Operator=atan
  Demux : Demux  Outputs=2
  Divide : Product  Inputs=/*
  angle : Outport
  wires:
  Divide/1 -> Atan/1
  Demux/2 -> Divide/2
  Demux/1 -> Divide/1
  Atan/1 -> Abs/1
  Abs/1 -> angle/1
  In1/1 -> Demux/1

== system Control_try/Team 1 Behaviour/Proximity_Finder_Ball ==
  In1 : Inport
  Demux : Demux  Outputs=2
  Sqrt : Sqrt  SaturateOnIntegerOverflow=on
  Square : Math  Operator=square  SaturateOnIntegerOverflow=on
  Square1 : Math  Operator=square  SaturateOnIntegerOverflow=on
  Sum : Sum
  DBR : Outport
  wires:
  In1/1 -> Demux/1
  Demux/1 -> Square/1
  Demux/2 -> Square1/1
  Square1/1 -> Sum/2
  Square/1 -> Sum/1
  Sum/1 -> Sqrt/1
  Sqrt/1 -> DBR/1

== system Control_try/Team 1 Behaviour/kick_direction ==
  In1 : Inport
  kick : Inport  Port=2
  Angle Finder1 : Subsystem
  Chart1 : Stateflow chart  TreatAsAtomicUnit=on
  Chart2 : Stateflow chart  TreatAsAtomicUnit=on
  Constant : Constant  Value=4
  Constant1 : Constant  Value=4
  Constant2 : Constant
  Cos : Trigonometry  Operator=cos
  Demux2 : Demux  Outputs=2
  Product : Product  Inputs=3
  Product1 : Product  Inputs=3
  Sin : Trigonometry
  Vector Concatenate : Concatenate  NumInputs=4
  Out1 : Outport
  wires:
  Demux2/2 -> Chart2/1(y)
  Demux2/1 -> Chart1/1(x)
  In1/1 -> Angle Finder1/1(In1), Demux2/1
  Chart1/1(Vx) -> Product/2
  Cos/1 -> Product/3
  Angle Finder1/1(angle) -> Cos/1, Sin/1
  Constant/1 -> Product/1
  Constant1/1 -> Product1/3
  Chart2/1(Vy) -> Product1/2
  Sin/1 -> Product1/1
  Product/1 -> Vector Concatenate/1
  Product1/1 -> Vector Concatenate/2
  Constant2/1 -> Vector Concatenate/3
  kick/1 -> Vector Concatenate/4
  Vector Concatenate/1 -> Out1/1

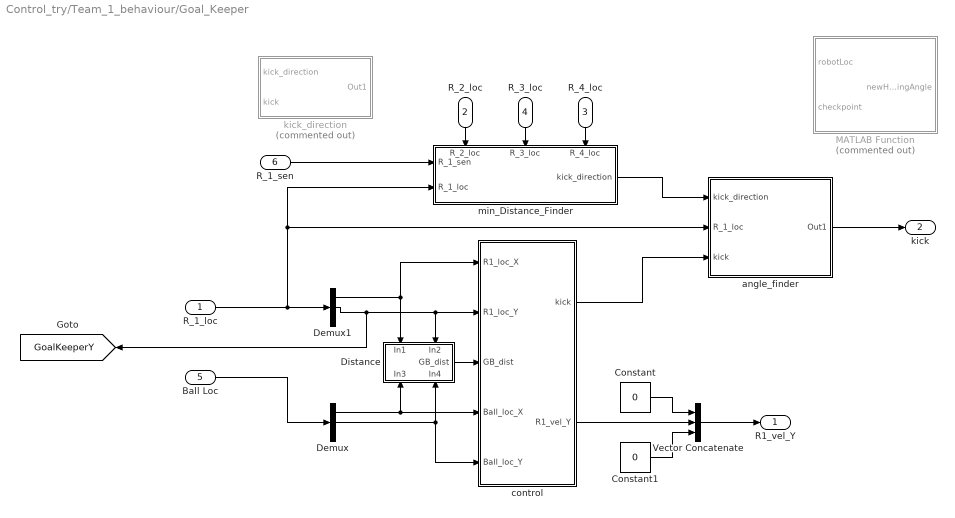
== system Control_try/Team_1_behaviour/Goal_Keeper ==
  R_1_loc : Inport
  R_2_loc : Inport  Port=2
  R_4_loc : Inport  Port=3
  R_3_loc : Inport  Port=4
  Ball Loc : Inport  Port=5
  R_1_sen : Inport  Port=6
  Constant : Constant  Value=0
  Constant1 : Constant  Value=0
  Demux : Demux  Outputs=3
  Demux1 : Demux  Outputs=3
  Distance : Subsystem
      settings: PortSchema="{\"entries\":[{\"content\":{\"sides\":[{\"content\":{\"connectorIds\":[]},\"type\":\"ConnectorPlacement.EquallySpacedRectSide\",\"uuid\":\"931fdb8b-3711-4e7f-9cbc-53e0dea53fca\"},{\"content\":{\"connectorIds\":[\"Out1\"],\"side\":\"RIGHT\"},\"type\":\"ConnectorPlacement.EquallySpacedRectSide\",\"uuid\":\"ee0c7800-c700-48d1-aa4f-dd4a30624bbc\"},{\"content\":{\"connectorIds\":[\"In1\",\"In2\"],\"side\":\"TOP\"},\"type\":\"ConnectorPlacement.EquallySpacedRectSide\",\"uuid\":\"9579cc4b-8b33-4755-9564-e19cfe104d2b\"},{\"content\":{\"connectorIds\":[\"In3\",\"In4\"],\"side\":\"BOTTOM\"},\"type\":\"ConnectorPlacement.EquallySpacedRectSide\",\"uuid\":\"3469c1a3-363b-4534-8624-9a42e1898f6f\"}]},\"type\":\"ConnectorPlacement.EquallySpacedConnector\",\"uuid\":\"efd995f2-e999-4310-9f3f-88c38333e880\"}],\"packageUris\":[\"http://schema.mathworks.com/mf0/Connector/R2020b\"],\"version\":\"1.0\"}"
  MATLAB Function : MATLAB Function  Commented=on  TreatAsAtomicUnit=on
  Vector Concatenate : Concatenate  NumInputs=3
  angle_finder : Subsystem
  control : Stateflow chart  TreatAsAtomicUnit=on
      settings: PortSchema="{\"entries\":[{\"content\":{\"sides\":[{\"content\":{\"connectorIds\":[\"In1\",\"In4\",\"In3\",\"In2\",\"In5\"]},\"type\":\"ConnectorPlacement.EquallySpacedRectSide\",\"uuid\":\"fa0fd246-e6b9-4dd4-94af-e6e1e45d6f7d\"},{\"content\":{\"connectorIds\":[\"Out1\",\"Out2\"],\"side\":\"RIGHT\"},\"type\":\"ConnectorPlacement.EquallySpacedRectSide\",\"uuid\":\"3f196244-96d1-41e4-aa84-a415e0f99109\"},{\"content\":{\"connectorIds\":[],\"side\":\"TOP\"},\"type\":\"ConnectorPlacement.EquallySpacedRectSide\",\"uuid\":\"731ebc3a-62ab-4275-8d10-19257bb8fb52\"}]},\"type\":\"ConnectorPlacement.EquallySpacedConnector\",\"uuid\":\"dccf28de-3df1-4952-8544-1d4b47a347e5\"}],\"packageUris\":[\"http://schema.mathworks.com/mf0/Connector/R2020b\"],\"version\":\"1.0\"}"
  kick_direction : Subsystem  Commented=on
  min_Distance_Finder : Subsystem
      settings: PortSchema="{\"entries\":[{\"content\":{\"sides\":[{\"content\":{\"connectorIds\":[\"In1\",\"In2\"]},\"type\":\"ConnectorPlacement.EquallySpacedRectSide\",\"uuid\":\"45cf91c7-7d38-4a19-bf35-d1d31095287a\"},{\"content\":{\"connectorIds\":[\"Out1\"],\"side\":\"RIGHT\"},\"type\":\"ConnectorPlacement.EquallySpacedRectSide\",\"uuid\":\"645394ba-2e5d-4060-b61c-cc9330ee0038\"},{\"content\":{\"connectorIds\":[\"In3\",\"In4\",\"In5\"],\"side\":\"TOP\"},\"type\":\"ConnectorPlacement.EquallySpacedRectSide\",\"uuid\":\"4fc56b73-04ec-476f-b487-f0e593f708ad\"},{\"content\":{\"connectorIds\":[],\"side\":\"BOTTOM\"},\"type\":\"ConnectorPlacement.EquallySpacedRectSide\",\"uuid\":\"cd306436-fd63-4e79-88e6-7a63c0840ed7\"}]},\"type\":\"ConnectorPlacement.EquallySpacedConnector\",\"uuid\":\"5cf2ee04-00eb-490b-958c-5fb90b43d325\"}],\"packageUris\":[\"http://schema.mathworks.com/mf0/Connector/R2020b\"],\"version\":\"1.0\"}"
  R1_vel_Y : Outport
  kick : Outport  Port=2
  tag scope: GoalKeeperY=global
  wires:
  Ball Loc/1 -> Demux/1
  Demux/2 -> control/5(Ball_loc_Y), Distance/4(In4)
  R_1_loc/1 -> Demux1/1, angle_finder/2(R_1_loc), min_Distance_Finder/2(R_1_loc)
  Demux1/2 -> [GoalKeeperY], control/4(R1_loc_Y), Distance/2(In2)
  Demux1/1 -> control/1(R1_loc_X), Distance/1(In1)
  R_2_loc/1 -> min_Distance_Finder/3(R_2_loc)
  R_3_loc/1 -> min_Distance_Finder/4(R_3_loc)
  R_4_loc/1 -> min_Distance_Finder/5(R_4_loc)
  R_1_sen/1 -> min_Distance_Finder/1(R_1_sen)
  Demux/1 -> control/2(Ball_loc_X), Distance/3(In3)
  control/2(R1_vel_Y) -> Vector Concatenate/2
  Distance/1(GB_dist) -> control/3(GB_dist)
  Vector Concatenate/1 -> R1_vel_Y/1
  Constant/1 -> Vector Concatenate/1
  Constant1/1 -> Vector Concatenate/3
  min_Distance_Finder/1(kick_direction) -> angle_finder/1(kick_direction)
  control/1(kick) -> angle_finder/3(kick)
  angle_finder/1(Out1) -> kick/1

== system Control_try/Team_1_behaviour/Goal_Keeper2 ==
  R_1_loc : Inport
  R_2_loc : Inport  Port=2
  R_4_loc : Inport  Port=3
  R_3_loc : Inport  Port=4
  Ball Loc : Inport  Port=5
  R_3_sen : Inport  Port=6
  Out1 : Outport
  Out2 : Outport  Port=2

== system Control_try/Team_1_behaviour/Goal_Keeper3 ==
  R_1_loc : Inport
  R_2_loc : Inport  Port=2
  R_4_loc : Inport  Port=3
  R_3_loc : Inport  Port=4
  Ball Loc : Inport  Port=5
  R_4_sen : Inport  Port=6
  Out1 : Outport
  Out2 : Outport  Port=2

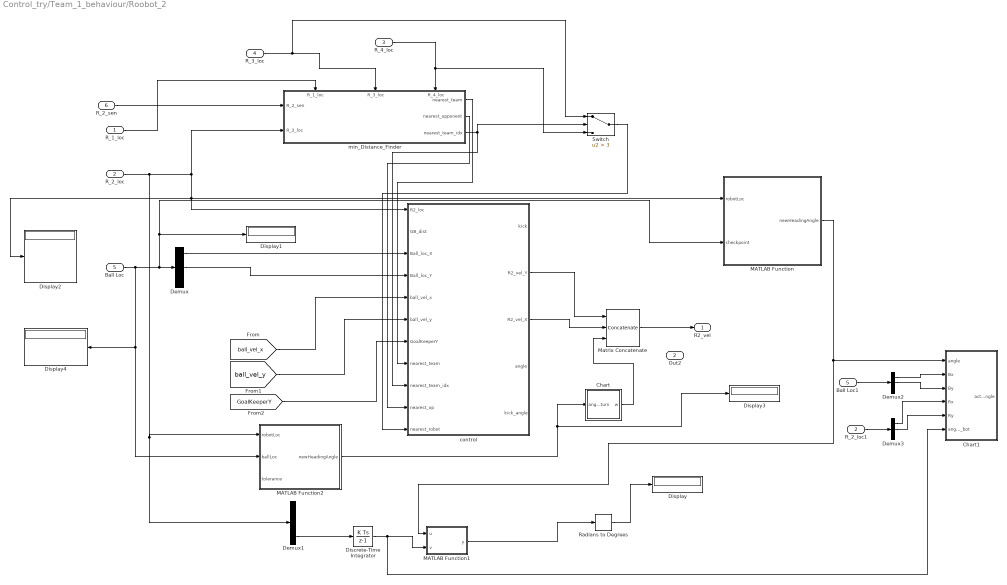
== system Control_try/Team_1_behaviour/Roobot_2 ==
  R_1_loc : Inport
  R_2_loc : Inport  Port=2
  R_4_loc : Inport  Port=3
  R_3_loc : Inport  Port=4
  Ball Loc : Inport  Port=5
  R_2_sen : Inport  Port=6
  Ball Loc1 : InportShadow  Port=5
  Chart : Stateflow chart  TreatAsAtomicUnit=on
  Chart1 : Stateflow chart  TreatAsAtomicUnit=on
      settings: PortSchema="{\"entries\":[{\"content\":{\"sides\":[{\"content\":{\"connectorIds\":[\"In5\",\"In1\",\"In2\",\"In3\",\"In4\",\"In6\"]},\"type\":\"ConnectorPlacement.EquallySpacedRectSide\",\"uuid\":\"cd25ea97-6441-4246-83f2-eec847899c89\"},{\"content\":{\"connectorIds\":[\"Out1\"],\"side\":\"RIGHT\"},\"type\":\"ConnectorPlacement.EquallySpacedRectSide\",\"uuid\":\"ef7d77a7-1549-4474-8b84-35bb8af5d0e7\"},{\"content\":{\"connectorIds\":[],\"side\":\"TOP\"},\"type\":\"ConnectorPlacement.EquallySpacedRectSide\",\"uuid\":\"0f0ce596-3061-42ac-890a-62bc4f21ac3e\"},{\"content\":{\"connectorIds\":[],\"side\":\"BOTTOM\"},\"type\":\"ConnectorPlacement.EquallySpacedRectSide\",\"uuid\":\"682b3de5-e999-4954-b7ff-f16ecbf9ea8f\"}]},\"type\":\"ConnectorPlacement.EquallySpacedConnector\",\"uuid\":\"15dca8e2-6a60-4a0d-80a5-3c295a61c828\"}],\"packageUris\":[\"http://schema.mathworks.com/mf0/Connector/R2020b\"],\"version\":\"1.0\"}"
  Demux{,1..3} (4 alike) : Demux  Outputs=3
  Discrete-Time Integrator : DiscreteIntegrator  SampleTime=-1  ICPrevOutput=DiscIntNeverNeededParam  ICPrevScaledInput=DiscIntNeverNeededParam
  Display{,1..4} (5 alike) : Display
  MATLAB Function : MATLAB Function  TreatAsAtomicUnit=on
  MATLAB Function1 : MATLAB Function  TreatAsAtomicUnit=on
  MATLAB Function2 : MATLAB Function  TreatAsAtomicUnit=on
  Matrix Concatenate : Concatenate  NumInputs=3  Mode=Multidimensional array
  R_2_loc1 : InportShadow  Port=2
  Radians to Degrees : simulink_extras/Transformations/Radians to Degrees
  Switch : Switch  Criteria=u2 > Threshold  Threshold=3
  control : Stateflow chart  TreatAsAtomicUnit=on
      settings: PortSchema="{\"entries\":[{\"content\":{\"sides\":[{\"content\":{\"connectorIds\":[\"In1\",\"In3\",\"In2\",\"In4\",\"In5\",\"In6\",\"In7\",\"In8\",\"In9\",\"In10\",\"In11\"]},\"type\":\"ConnectorPlacement.EquallySpacedRectSide\",\"uuid\":\"fa0fd246-e6b9-4dd4-94af-e6e1e45d6f7d\"},{\"content\":{\"connectorIds\":[\"Out1\",\"Out2\",\"Out3\",\"Out5\",\"Out4\"],\"side\":\"RIGHT\"},\"type\":\"ConnectorPlacement.EquallySpacedRectSide\",\"uuid\":\"3f196244-96d1-41e4-aa84-a415e0f99109\"},{\"content\":{\"connectorIds\":[],\"side\":\"TOP\"},\"type\":\"ConnectorPlacement.EquallySpacedRectSide\",\"uuid\":\"731ebc3a-62ab-4275-8d10-19257bb8fb52\"}]},\"type\":\"ConnectorPlacement.EquallySpacedConnector\",\"uuid\":\"dccf28de-3df1-4952-8544-1d4b47a347e5\"}],\"packageUris\":[\"http://schema.mathworks.com/mf0/Connector/R2020b\"],\"version\":\"1.0\"}"
  min_Distance_Finder : Subsystem
      settings: PortSchema="{\"entries\":[{\"content\":{\"sides\":[{\"content\":{\"connectorIds\":[\"In1\",\"In2\"]},\"type\":\"ConnectorPlacement.EquallySpacedRectSide\",\"uuid\":\"45cf91c7-7d38-4a19-bf35-d1d31095287a\"},{\"content\":{\"connectorIds\":[\"Out1\",\"Out2\",\"Out3\"],\"side\":\"RIGHT\"},\"type\":\"ConnectorPlacement.EquallySpacedRectSide\",\"uuid\":\"645394ba-2e5d-4060-b61c-cc9330ee0038\"},{\"content\":{\"connectorIds\":[\"In3\",\"In4\",\"In5\"],\"side\":\"TOP\"},\"type\":\"ConnectorPlacement.EquallySpacedRectSide\",\"uuid\":\"4fc56b73-04ec-476f-b487-f0e593f708ad\"},{\"content\":{\"connectorIds\":[],\"side\":\"BOTTOM\"},\"type\":\"ConnectorPlacement.EquallySpacedRectSide\",\"uuid\":\"cd306436-fd63-4e79-88e6-7a63c0840ed7\"}]},\"type\":\"ConnectorPlacement.EquallySpacedConnector\",\"uuid\":\"5cf2ee04-00eb-490b-958c-5fb90b43d325\"}],\"packageUris\":[\"http://schema.mathworks.com/mf0/Connector/R2020b\"],\"version\":\"1.0\"}"
  R2_vel : Outport
  Out2 : Outport  Port=2
  wires:
  [ball_vel_x] -> control/5(ball_vel_x)
  [ball_vel_y] -> control/6(ball_vel_y)
  [GoalKeeperY] -> control/7(GoalKeeperY)
  R_2_loc/1 -> min_Distance_Finder/2(R_2_loc), Display2/1, MATLAB Function/1(robotLoc), control/1(R2_loc), MATLAB Function2/1(robotLoc), Demux1/1
  R_2_sen/1 -> min_Distance_Finder/1(R_2_sen)
  R_4_loc/1 -> Switch/3, min_Distance_Finder/5(R_4_loc)
  R_3_loc/1 -> Switch/1, min_Distance_Finder/4(R_3_loc)
  R_1_loc/1 -> min_Distance_Finder/3(R_1_loc)
  Ball Loc/1 -> Display4/1, MATLAB Function2/2(ballLoc), MATLAB Function/2(checkpoint), Display1/1, Demux/1
  Demux/1 -> control/2(Ball_loc_X)
  Demux/2 -> control/4(Ball_loc_Y)
  min_Distance_Finder/3(nearest_team_idx) -> control/9(nearest_team_idx), Switch/2
  min_Distance_Finder/2(nearest_opponent) -> control/10(nearest_op)
  min_Distance_Finder/1(nearest_team) -> control/8(nearest_team)
  Switch/1 -> control/11(nearest_robot)
  control/2(R2_vel_Y) -> Matrix Concatenate/1
  control/3(R2_vel_X) -> Matrix Concatenate/2
  Matrix Concatenate/1 -> R2_vel/1
  Chart/1(w) -> Matrix Concatenate/3
  MATLAB Function/1(newHeadingAngle) -> Chart1/5(angle), MATLAB Function1/1(u)
  Demux1/3 -> Discrete-Time Integrator/1
  Discrete-Time Integrator/1 -> Chart1/6(angle_bot), MATLAB Function1/2(v)
  MATLAB Function1/1(y) -> Radians to Degrees/1
  Radians to Degrees/1 -> Display/1
  Ball Loc1/1 -> Demux2/1
  Demux2/1 -> Chart1/1(Bx)
  Demux2/2 -> Chart1/2(By)
  R_2_loc1/1 -> Demux3/1
  Demux3/1 -> Chart1/3(Rx)
  Demux3/2 -> Chart1/4(Ry)
  MATLAB Function2/1(newHeadingAngle) -> Display3/1, Chart/1(angle_to_turn)

== system Control_try/Team 1 Behaviour/kick_direction/Angle Finder1 ==
  In1 : Inport
  Abs : Abs
  Atan : Trigonometry  Operator=atan
  Demux : Demux  Outputs=2
  Divide : Product  Inputs=/*
  angle : Outport
  wires:
  Divide/1 -> Atan/1
  Demux/2 -> Divide/2
  Demux/1 -> Divide/1
  Atan/1 -> Abs/1
  Abs/1 -> angle/1
  In1/1 -> Demux/1

== system Control_try/Team_1_behaviour/Goal_Keeper/Distance ==
  In1 : Inport
  In2 : Inport  Port=2
  In3 : Inport  Port=3
  In4 : Inport  Port=4
  Square : Math  Operator=square  SaturateOnIntegerOverflow=on
  Square Root : Sqrt  SaturateOnIntegerOverflow=on
  Square1 : Math  Operator=square  SaturateOnIntegerOverflow=on
  Sum : Sum  Inputs=|+-
  Sum1 : Sum  Inputs=|+-
  Sum2 : Sum  Inputs=|++
  GB_dist : Outport
  wires:
  Square1/1 -> Sum2/2
  Sum2/1 -> Square Root/1
  Square/1 -> Sum2/1
  Sum1/1 -> Square1/1
  Sum/1 -> Square/1
  In1/1 -> Sum/1
  In3/1 -> Sum/2
  In2/1 -> Sum1/1
  In4/1 -> Sum1/2
  Square Root/1 -> GB_dist/1

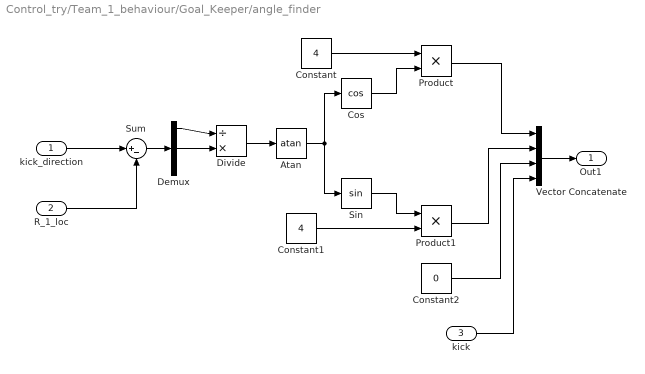
== system Control_try/Team_1_behaviour/Goal_Keeper/angle_finder ==
  kick_direction : Inport
  R_1_loc : Inport  Port=2
  kick : Inport  Port=3
  Atan : Trigonometry  Operator=atan
  Constant : Constant  Value=4
  Constant1 : Constant  Value=4
  Constant2 : Constant  Value=0
  Cos : Trigonometry  Operator=cos
  Demux : Demux  Outputs=3
  Divide : Product  Inputs=/*
  Product : Product
  Product1 : Product
  Sin : Trigonometry
  Sum : Sum  Inputs=|+-
  Vector Concatenate : Concatenate  NumInputs=4
  Out1 : Outport
  wires:
  kick_direction/1 -> Sum/1
  R_1_loc/1 -> Sum/2
  Sum/1 -> Demux/1
  Demux/1 -> Divide/1
  Demux/2 -> Divide/2
  Divide/1 -> Atan/1
  Atan/1 -> Cos/1, Sin/1
  Constant/1 -> Product/1
  Cos/1 -> Product/2
  Sin/1 -> Product1/1
  Constant1/1 -> Product1/2
  Vector Concatenate/1 -> Out1/1
  kick/1 -> Vector Concatenate/4
  Constant2/1 -> Vector Concatenate/3
  Product1/1 -> Vector Concatenate/2
  Product/1 -> Vector Concatenate/1

== system Control_try/Team_1_behaviour/Goal_Keeper/kick_direction ==
  kick_direction : Inport
  kick : Inport  Port=2
  Angle Finder1 : Subsystem
  Chart1 : Stateflow chart  TreatAsAtomicUnit=on
  Chart2 : Stateflow chart  TreatAsAtomicUnit=on
  Constant : Constant  Value=4
  Constant1 : Constant  Value=4
  Constant2 : Constant  Value=0
  Cos : Trigonometry  Operator=cos
  Demux2 : Demux  Outputs=3
  Product : Product  Inputs=3
  Product1 : Product  Inputs=3
  Sin : Trigonometry
  Vector Concatenate : Concatenate  NumInputs=4
  Vector Concatenate1 : Concatenate
  Out1 : Outport
  wires:
  Demux2/2 -> Vector Concatenate1/2, Chart2/1(y)
  Demux2/1 -> Vector Concatenate1/1, Chart1/1(x)
  kick_direction/1 -> Demux2/1
  Chart1/1(Vx) -> Product/2
  Cos/1 -> Product/3
  Angle Finder1/1(angle) -> Cos/1, Sin/1
  Constant/1 -> Product/1
  Constant1/1 -> Product1/3
  Chart2/1(Vy) -> Product1/2
  Sin/1 -> Product1/1
  Product/1 -> Vector Concatenate/1
  Product1/1 -> Vector Concatenate/2
  Constant2/1 -> Vector Concatenate/3
  kick/1 -> Vector Concatenate/4
  Vector Concatenate/1 -> Out1/1
  Vector Concatenate1/1 -> Angle Finder1/1(In1)

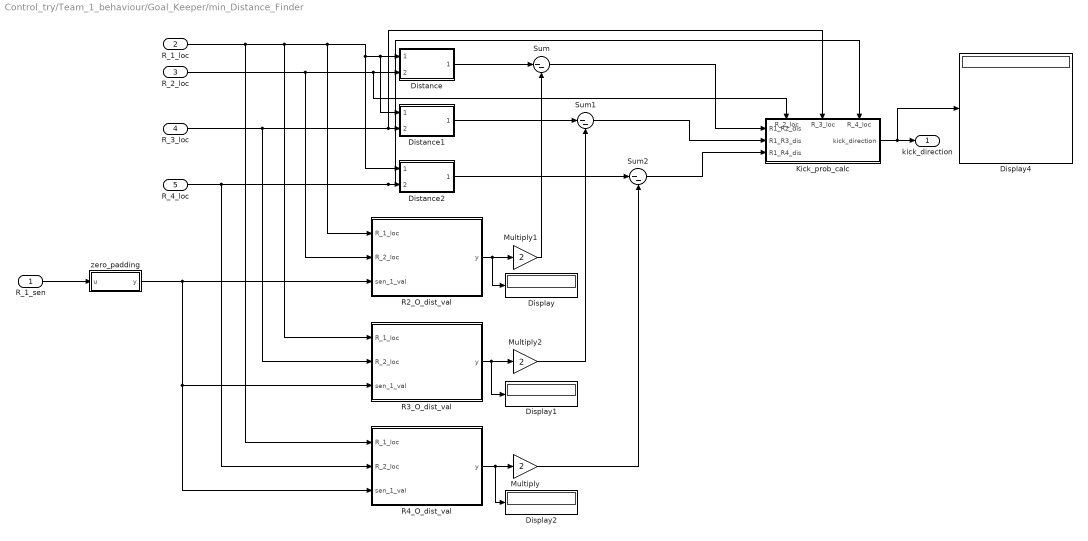
== system Control_try/Team_1_behaviour/Goal_Keeper/min_Distance_Finder ==
  R_1_sen : Inport
  R_1_loc : Inport  Port=2
  R_2_loc : Inport  Port=3
  R_3_loc : Inport  Port=4
  R_4_loc : Inport  Port=5
  Display{,1..2,4} (4 alike) : Display
  Distance : Subsystem
  Distance1 : Subsystem
  Distance2 : Subsystem
  Kick_prob_calc : Stateflow chart  TreatAsAtomicUnit=on
      settings: PortSchema="{\"entries\":[{\"content\":{\"sides\":[{\"content\":{\"connectorIds\":[\"In4\",\"In5\",\"In6\"]},\"type\":\"ConnectorPlacement.EquallySpacedRectSide\",\"uuid\":\"64545375-395a-4478-8a53-b77c7ccd5016\"},{\"content\":{\"connectorIds\":[\"Out1\"],\"side\":\"RIGHT\"},\"type\":\"ConnectorPlacement.EquallySpacedRectSide\",\"uuid\":\"7cc0c28a-cc26-4f23-9952-6261e736221a\"},{\"content\":{\"connectorIds\":[\"In2\",\"In3\",\"In1\"],\"side\":\"TOP\"},\"type\":\"ConnectorPlacement.EquallySpacedRectSide\",\"uuid\":\"3f39c863-1804-4707-87c1-6f77798d874b\"},{\"content\":{\"connectorIds\":[],\"side\":\"BOTTOM\"},\"type\":\"ConnectorPlacement.EquallySpacedRectSide\",\"uuid\":\"dd00a5df-2ac1-49a5-bc9d-cbc3bc53305b\"}]},\"type\":\"ConnectorPlacement.EquallySpacedConnector\",\"uuid\":\"731ad359-9b43-4c19-839e-d6f1a372c8a6\"}],\"packageUris\":[\"http://schema.mathworks.com/mf0/Connector/R2020b\"],\"version\":\"1.0\"}"
  Multiply : Gain  Gain=2
  Multiply1 : Gain  Gain=2
  Multiply2 : Gain  Gain=2
  R2_O_dist_val : Subsystem
  R3_O_dist_val : Subsystem
  R4_O_dist_val : Subsystem
  Sum : Sum  Inputs=|--
  Sum1 : Sum  Inputs=|--
  Sum2 : Sum  Inputs=|--
  zero_padding : MATLAB Function  TreatAsAtomicUnit=on
  kick_direction : Outport
  wires:
  R_2_loc/1 -> R2_O_dist_val/2(R_2_loc), Distance/2(R_2_loc), Kick_prob_calc/2(R_2_loc)
  R_1_loc/1 -> R4_O_dist_val/1(R_1_loc), R3_O_dist_val/1(R_1_loc), R2_O_dist_val/1(R_1_loc), Distance2/1(R_1_loc), Distance1/1(R_1_loc), Distance/1(R_1_loc)
  R_3_loc/1 -> R3_O_dist_val/2(R_2_loc), Distance1/2(R_3_loc), Kick_prob_calc/3(R_3_loc)
  R_4_loc/1 -> R4_O_dist_val/2(R_2_loc), Distance2/2(R_4_loc), Kick_prob_calc/1(R_4_loc)
  Kick_prob_calc/1(kick_direction) -> Display4/1, kick_direction/1
  R_1_sen/1 -> zero_padding/1(u)
  zero_padding/1(y) -> R3_O_dist_val/3(sen_1_val), R4_O_dist_val/3(sen_1_val), R2_O_dist_val/3(sen_1_val)
  R2_O_dist_val/1(y) -> Display/1, Multiply1/1
  R3_O_dist_val/1(y) -> Display1/1, Multiply2/1
  R4_O_dist_val/1(y) -> Display2/1, Multiply/1
  Distance/1(R1_R2_dis) -> Sum/1
  Multiply1/1 -> Sum/2
  Distance1/1(R1_R3_dis) -> Sum1/1
  Distance2/1(R1_R4_dis) -> Sum2/1
  Multiply2/1 -> Sum1/2
  Multiply/1 -> Sum2/2
  Sum/1 -> Kick_prob_calc/4(R1_R2_dis)
  Sum1/1 -> Kick_prob_calc/5(R1_R3_dis)
  Sum2/1 -> Kick_prob_calc/6(R1_R4_dis)

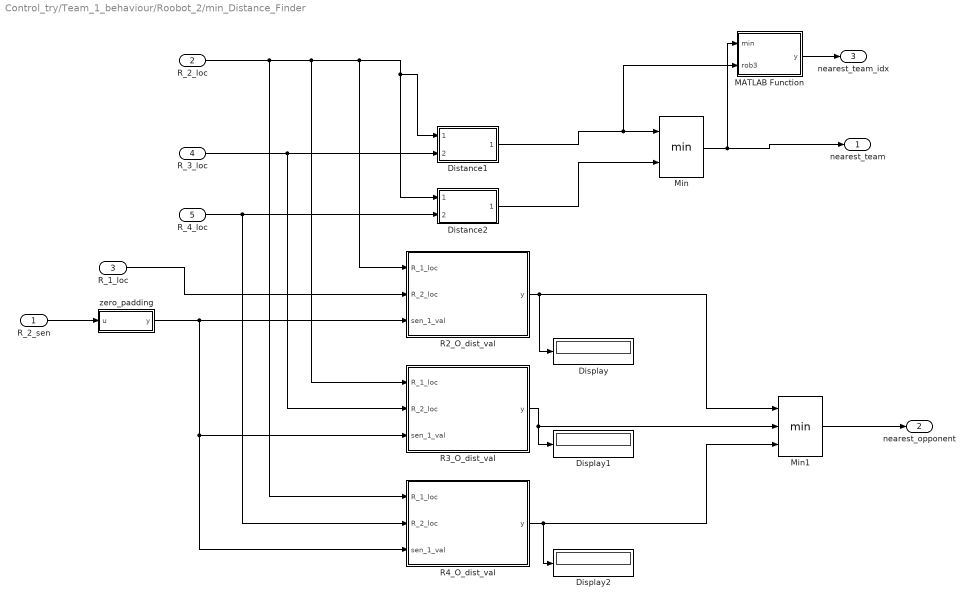
== system Control_try/Team_1_behaviour/Roobot_2/min_Distance_Finder ==
  R_2_sen : Inport
  R_2_loc : Inport  Port=2
  R_1_loc : Inport  Port=3
  R_3_loc : Inport  Port=4
  R_4_loc : Inport  Port=5
  Display : Display
  Display1 : Display
  Display2 : Display
  Distance1 : Subsystem
  Distance2 : Subsystem
  MATLAB Function : MATLAB Function  TreatAsAtomicUnit=on
  Min : MinMax  Inputs=2
  Min1 : MinMax  Inputs=3
  R2_O_dist_val : Subsystem
  R3_O_dist_val : Subsystem
  R4_O_dist_val : Subsystem
  zero_padding : MATLAB Function  TreatAsAtomicUnit=on
  nearest_team : Outport
  nearest_opponent : Outport  Port=2
  nearest_team_idx : Outport  Port=3
  wires:
  R_1_loc/1 -> R2_O_dist_val/2(R_2_loc)
  R_2_loc/1 -> R4_O_dist_val/1(R_1_loc), R3_O_dist_val/1(R_1_loc), R2_O_dist_val/1(R_1_loc), Distance2/1(R_1_loc), Distance1/1(R_1_loc)
  R_3_loc/1 -> R3_O_dist_val/2(R_2_loc), Distance1/2(R_3_loc)
  R_4_loc/1 -> R4_O_dist_val/2(R_2_loc), Distance2/2(R_4_loc)
  R_2_sen/1 -> zero_padding/1(u)
  zero_padding/1(y) -> R3_O_dist_val/3(sen_1_val), R4_O_dist_val/3(sen_1_val), R2_O_dist_val/3(sen_1_val)
  R2_O_dist_val/1(y) -> Min1/1, Display/1
  R3_O_dist_val/1(y) -> Min1/2, Display1/1
  R4_O_dist_val/1(y) -> Min1/3, Display2/1
  Min/1 -> MATLAB Function/1(min), nearest_team/1
  Min1/1 -> nearest_opponent/1
  Distance1/1(R1_R3_dis) -> MATLAB Function/2(rob3), Min/1
  Distance2/1(R1_R4_dis) -> Min/2
  MATLAB Function/1(y) -> nearest_team_idx/1

== system Control_try/Team_1_behaviour/Goal_Keeper/kick_direction/Angle Finder1 ==
  In1 : Inport
  Abs : Abs
  Atan : Trigonometry  Operator=atan
  Demux : Demux  Outputs=2
  Divide : Product  Inputs=/*
  angle : Outport
  wires:
  Divide/1 -> Atan/1
  Demux/2 -> Divide/2
  Demux/1 -> Divide/1
  Atan/1 -> Abs/1
  Abs/1 -> angle/1
  In1/1 -> Demux/1
